simulink model "DC"  (R2023a)
settings: Solver=VariableStepAuto  StartTime=0.0  StopTime=1  RelTol=1e-3
undefined symbols (not defined in the file or in its folder): B1, J1, Kb1, Kt1, L1, R1
settings Model: Creator=Hi  LastModifiedBy=Hi

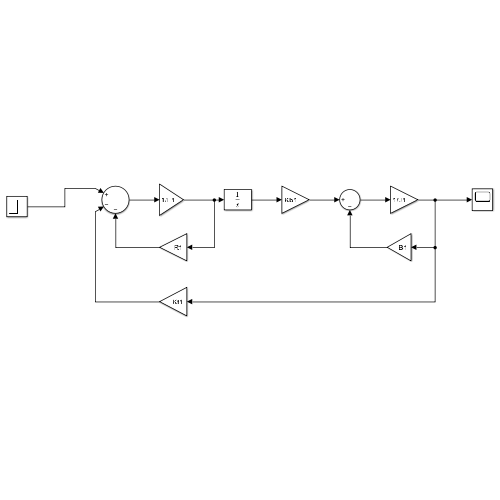
[thumbnail: Simulink's stored preview of the top-level diagram]
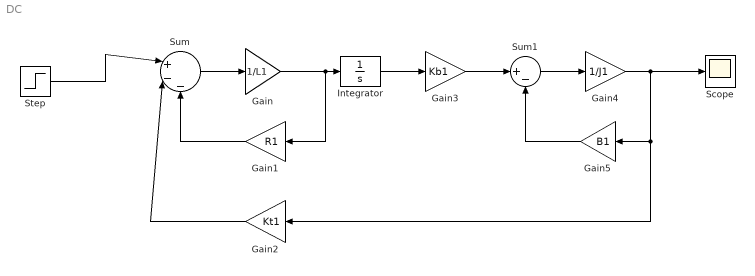
== system DC ==
  Gain : Gain  Gain=1/L1
  Gain1 : Gain  Gain=R1
  Gain2 : Gain  Gain=Kt1
  Gain3 : Gain  Gain=Kb1
  Gain4 : Gain  Gain=1/J1
  Gain5 : Gain  Gain=B1
  Integrator : Integrator
  Scope : Scope
  Step : Step  SampleTime=0
  Sum : Sum  Inputs=|+--  OutDataTypeStr=Inherit: Keep LSB
  Sum1 : Sum  Inputs=|+-
  wires:
  Sum1/1 -> Gain4/1
  Sum/1 -> Gain/1
  Gain5/1 -> Sum1/2
  Integrator/1 -> Gain3/1
  Gain3/1 -> Sum1/1
  Gain1/1 -> Sum/3
  Gain2/1 -> Sum/2
  Gain/1 -> Integrator/1, Gain1/1
  Gain4/1 -> Scope/1, Gain5/1, Gain2/1
  Step/1 -> Sum/1
